simulink model "ARP_01_lib_TruthTables"  (R2014a)
settings: Solver=ode45  StartTime=0.0  StopTime=10.0  RelTol=1e-3
(part 2 of 2)

== stateflow chart ARP_01_lib_TruthTables/Chart ==
  note: num of bmlID=2
  note: num of bmlID=2
  note: num of bmlID=2
  note: num of sbmID=4
  note: num of bmlID=18
  note: num of bmlID=3
  note: num of bmlID=18
  note: num of bmlID=18
      | 17=neutralHead
      | 18=onceBlink
  note: num of bmlID=2
  note: num of bmlID=8
  note: num of bmlID=8
  data: bmlID function_input double; poseBML function_output double size=[256,1]; bmlID function_input double; poseBML function_output double size=[256,1]; bmlID function_input double; poseBML function_output double size=[256,1]; bmlID function_input double; poseBML function_output double size=[256,1]; bmlID function_input double; poseBML function_output double size=[256,1]; sbmID function_input double; poseSBM function_output double size=[256,1]; sbmID function_input double; poseSBM function_output double size=[256,1]; bmlID function_input double; poseBML function_output double size=[256,1]; bmlID function_input double; poseBML function_output double size=[256,1]; bmlID function_input double; poseBML function_output double size=[256,1]; bmlID function_input double; poseBML function_output double size=[256,1]; bmlID function_input double; gazeBML function_output double size=[256,1]; bmlID function_input double; gazeBML function_output double size=[256,1]; bmlID function_input double; poseBML function_output double size=[256,1]; bmlID function_input double; poseBML function_output double size=[256,1]; bmlID function_input double size=1; poseBML function_output double size=[256,1]; sbmID function_input double; poseSBM function_output double size=[256,1]; bmlID function_input double; poseBML function_output double size=[256,1]; bmlID function_input double; gazeBML function_output double size=[256,1]
  function poseBML = rockPoseTable(bmlID):
    | function poseBML = rockPoseTable(bmlID)
    | 
    | aVarTruthTableCondition_1 = false;
    | aVarTruthTableCondition_2 = false;
    | 
    | 
    | % rock
    | 
    | aVarTruthTableCondition_1 = logical(bmlID==1);
    | 
    | % rock
    | 
    | aVarTruthTableCondition_2 = logical(bmlID==2);
    | 
    | if (aVarTruthTableCondition_1)
    |     aFcnTruthTableAction_1();
    | elseif (aVarTruthTableCondition_2)
    |     aFcnTruthTableAction_2();
    | else % Default
    |     aFcnTruthTableAction_1();
    | end
    | 
    | function aFcnTruthTableAction_1()
    | 
    | % rock
    | 
    | poseBML=encStr2Arr('<?xml version="1.0" ?><act><bml><animation name="ChrBrad@Idle01_BeatFistMidLf02"/></bml></act>');
    | 
    | function aFcnTruthTableAction_2()
    | 
    | % rock2
    | 
    | poseBML=encStr2Arr('<?xml version="1.0" ?><act><bml><animation name="ChrBrad@Idle01_BeatFistMidLf01"/></bml></act>');
  function poseBML = paperPoseBradTable(bmlID):
    | function poseBML = paperPoseBradTable(bmlID)
    | 
    | aVarTruthTableCondition_1 = false;
    | aVarTruthTableCondition_2 = false;
    | 
    | 
    | % paper
    | 
    | aVarTruthTableCondition_1 = logical(bmlID==1);
    | 
    | % paper2
    | 
    | aVarTruthTableCondition_2 = logical(bmlID==2);
    | 
    | if (aVarTruthTableCondition_1)
    |     aFcnTruthTableAction_1();
    | elseif (aVarTruthTableCondition_2)
    |     aFcnTruthTableAction_2();
    | else % Default
    |     aFcnTruthTableAction_2();
    | end
    | 
    | function aFcnTruthTableAction_1()
    | 
    | % paper
    | 
    | poseBML=encStr2Arr('<?xml version="1.0" ?><act><bml><animation name="ChrBrad@Idle01_OfferLf01"/></bml></act>');
    | 
    | function aFcnTruthTableAction_2()
    | 
    | % paper2
    | 
    | poseBML=encStr2Arr('<?xml version="1.0" ?><act><bml><animation name="ChrBrad@Idle01_YouLf01"/></bml></act>');
  function poseBML = paperPoseRachelTable(bmlID):
    | function poseBML = paperPoseRachelTable(bmlID)
    | 
    | aVarTruthTableCondition_1 = false;
    | 
    | 
    | % paper
    | 
    | aVarTruthTableCondition_1 = logical(bmlID==1);
    | 
    | if (aVarTruthTableCondition_1)
    |     aFcnTruthTableAction_1();
    | else % Default
    |     aFcnTruthTableAction_1();
    | end
    | 
    | function aFcnTruthTableAction_1()
    | 
    | % paper
    | 
    | poseBML=encStr2Arr('<?xml version="1.0" ?><act><bml><animation name="ChrBrad@Idle01_YouLf01"/></bml></act>');
  function poseBML = scissorsPoseBradTable(bmlID):
    | function poseBML = scissorsPoseBradTable(bmlID)
    | 
    | aVarTruthTableCondition_1 = false;
    | aVarTruthTableCondition_2 = false;
    | 
    | 
    | % scissors
    | 
    | aVarTruthTableCondition_1 = logical(bmlID==1);
    | 
    | % scissors2
    | 
    | aVarTruthTableCondition_2 = logical(bmlID==2);
    | 
    | if (aVarTruthTableCondition_1)
    |     aFcnTruthTableAction_1();
    | elseif (aVarTruthTableCondition_2)
    |     aFcnTruthTableAction_2();
    | else % Default
    |     aFcnTruthTableAction_1();
    | end
    | 
    | function aFcnTruthTableAction_1()
    | 
    | % scissors
    | 
    | poseBML=encStr2Arr('<?xml version="1.0" ?><act><bml><animation name="ChrBrad@Idle01_YouLf01"/></bml></act>');
    | 
    | function aFcnTruthTableAction_2()
    | 
    | % scissors2
    | 
    | poseBML=encStr2Arr('<?xml version="1.0" ?><act><bml><animation name="ChrBrad@Idle01_OfferLf01"/></bml></act>');
  function poseBML = scissorsPoseRachelTable(bmlID):
    | function poseBML = scissorsPoseRachelTable(bmlID)
    | 
    | aVarTruthTableCondition_1 = false;
    | 
    | 
    | % scissors
    | 
    | aVarTruthTableCondition_1 = logical(bmlID==1);
    | 
    | if (aVarTruthTableCondition_1)
    |     aFcnTruthTableAction_1();
    | else % Default
    |     aFcnTruthTableAction_1();
    | end
    | 
    | function aFcnTruthTableAction_1()
    | 
    | % scissors
    | 
    | poseBML=encStr2Arr('<?xml version="1.0" ?><act><bml><animation name="ChrBrad@Idle01_YouLf01"/></bml></act>');
  function poseSBM = handPoseSBTable(sbmID):
    | function poseSBM = handPoseSBTable(sbmID)
    | 
    | aVarTruthTableCondition_1 = false;
    | aVarTruthTableCondition_2 = false;
    | aVarTruthTableCondition_3 = false;
    | aVarTruthTableCondition_4 = false;
    | 
    | 
    | % fingersClose
    | 
    | aVarTruthTableCondition_1 = logical(sbmID==1);
    | 
    | % fingersNeutral
    | 
    | aVarTruthTableCondition_2 = logical(sbmID==2);
    | 
    | % lshoulkderForward
    | 
    | aVarTruthTableCondition_3 = logical(sbmID==3);
    | 
    | % lshoulkderNeutral
    | 
    | aVarTruthTableCondition_4 = logical(sbmID==4);
    | 
    | if (aVarTruthTableCondition_1)
    |     aFcnTruthTableAction_1();
    | elseif (aVarTruthTableCondition_2)
    |     aFcnTruthTableAction_2();
    | elseif (aVarTruthTableCondition_3)
    |     aFcnTruthTableAction_3();
    | elseif (aVarTruthTableCondition_4)
    |     aFcnTruthTableAction_4();
    | else % Default
    |     aFcnTruthTableAction_1();
    | end
    | 
    | function aFcnTruthTableAction_1()
    | 
    | % fingersClose
    | 
    | poseSBM=encStr2Arr('brad.getSkeleton().getJointByName("l_pinky1").setPostrotation(SrQuat(1,0,0,0.5)); brad.getSkeleton().getJointByName("l_ring1").setPostrotation(SrQuat(1,0,0,0.5))');
    | 
    | function aFcnTruthTableAction_2()
    | 
    | % fingersNeutral
    | 
    | poseSBM=encStr2Arr('brad.getSkeleton().getJointByName("l_pinky1").setPostrotation(SrQuat(1,0,0,0)); brad.getSkeleton().getJointByName("l_ring1").setPostrotation(SrQuat(1,0,0,0))');
    | 
    | function aFcnTruthTableAction_3()
    | 
    | % lshoulkderForward
    | 
    | poseSBM=encStr2Arr('brad.getSkeleton().getJointByName("l_sternoclavicular").setPostrotation(SrQuat(1,0,0,0.05))');
    | 
    | function aFcnTruthTableAction_4()
    | 
    | % lshoulkderNeutral
    | 
    | poseSBM=encStr2Arr('brad.getSkeleton().getJointByName("l_sternoclavicular").setPostrotation(SrQuat(1,0,0,0))');
  function poseSBM = handPoseSBRachelTable(sbmID):
    | function poseSBM = handPoseSBRachelTable(sbmID)
    | 
    | aVarTruthTableCondition_1 = false;
    | aVarTruthTableCondition_2 = false;
    | aVarTruthTableCondition_3 = false;
    | aVarTruthTableCondition_4 = false;
    | 
    | 
    | % fingersClose
    | 
    | aVarTruthTableCondition_1 = logical(sbmID==1);
    | 
    | % fingersNeutral
    | 
    | aVarTruthTableCondition_2 = logical(sbmID==2);
    | 
    | % lshoulkderForward
    | 
    | aVarTruthTableCondition_3 = logical(sbmID==3);
    | 
    | % lshoulkderNeutral
    | 
    | aVarTruthTableCondition_4 = logical(sbmID==4);
    | 
    | if (aVarTruthTableCondition_1)
    |     aFcnTruthTableAction_1();
    | elseif (aVarTruthTableCondition_2)
    |     aFcnTruthTableAction_2();
    | elseif (aVarTruthTableCondition_3)
    |     aFcnTruthTableAction_3();
    | elseif (aVarTruthTableCondition_4)
    |     aFcnTruthTableAction_4();
    | else % Default
    |     aFcnTruthTableAction_1();
    | end
    | 
    | function aFcnTruthTableAction_1()
    | 
    | % fingersClose
    | 
    | poseSBM=encStr2Arr('Rachel.getSkeleton().getJointByName("l_pinky1").setPostrotation(SrQuat(1,0,0,0.5)); Rachel.getSkeleton().getJointByName("l_ring1").setPostrotation(SrQuat(1,0,0,0.5))');
    | 
    | function aFcnTruthTableAction_2()
    | 
    | % fingersNeutral
    | 
    | poseSBM=encStr2Arr('Rachel.getSkeleton().getJointByName("l_pinky1").setPostrotation(SrQuat(1,0,0,0)); Rachel.getSkeleton().getJointByName("l_ring1").setPostrotation(SrQuat(1,0,0,0))');
    | 
    | function aFcnTruthTableAction_3()
    | 
    | % lshoulkderForward
    | 
    | poseSBM=encStr2Arr('Rachel.getSkeleton().getJointByName("l_sternoclavicular").setPostrotation(SrQuat(1,0,0,0.05))');
    | 
    | function aFcnTruthTableAction_4()
    | 
    | % lshoulkderNeutral
    | 
    | poseSBM=encStr2Arr('Rachel.getSkeleton().getJointByName("l_sternoclavicular").setPostrotation(SrQuat(1,0,0,0))');
  function poseBML=idlePoseBradTable(bmlID):
    | function poseBML=idlePoseBradTable(bmlID)
    | 
    | aVarTruthTableCondition_1 = false;
    | aVarTruthTableCondition_2 = false;
    | aVarTruthTableCondition_3 = false;
    | aVarTruthTableCondition_4 = false;
    | aVarTruthTableCondition_5 = false;
    | aVarTruthTableCondition_6 = false;
    | aVarTruthTableCondition_7 = false;
    | aVarTruthTableCondition_8 = false;
    | aVarTruthTableCondition_9 = false;
    | aVarTruthTableCondition_10 = false;
    | aVarTruthTableCondition_11 = false;
    | aVarTruthTableCondition_12 = false;
    | aVarTruthTableCondition_13 = false;
    | aVarTruthTableCondition_14 = false;
    | aVarTruthTableCondition_15 = false;
    | aVarTruthTableCondition_16 = false;
    | aVarTruthTableCondition_17 = false;
    | aVarTruthTableCondition_18 = false;
    | 
    | 
    | 
    | aVarTruthTableCondition_1 = logical(bmlID==1);
    | 
    | 
    | aVarTruthTableCondition_2 = logical(bmlID==2);
    | 
    | 
    | aVarTruthTableCondition_3 = logical(bmlID==3);
    | 
    | 
    | aVarTruthTableCondition_4 = logical(bmlID==4);
    | 
    | 
    | aVarTruthTableCondition_5 = logical(bmlID==5);
    | 
    | 
    | aVarTruthTableCondition_6 = logical(bmlID==6);
    | 
    | 
    | aVarTruthTableCondition_7 = logical(bmlID==7);
    | 
    | 
    | aVarTruthTableCondition_8 = logical(bmlID==8);
    | 
    | 
    | aVarTruthTableCondition_9 = logical(bmlID==9);
    | 
    | 
    | aVarTruthTableCondition_10 = logical(bmlID==10);
    | 
    | 
    | aVarTruthTableCondition_11 = logical(bmlID==11);
    | 
    | 
    | aVarTruthTableCondition_12 = logical(bmlID==12);
    | 
    | 
    | aVarTruthTableCondition_13 = logical(bmlID==13);
    | 
    | 
    | aVarTruthTableCondition_14 = logical(bmlID==14);
    | 
    | 
    | aVarTruthTableCondition_15 = logical(bmlID==15);
    | 
    | 
    | aVarTruthTableCondition_16 = logical(bmlID==16);
    | 
    | 
    | aVarTruthTableCondition_17 = logical(bmlID==17);
    | 
    | 
    | aVarTruthTableCondition_18 = logical(bmlID==18);
    | 
    | if (aVarTruthTableCondition_1)
    |     aFcnTruthTableAction_1();
    | elseif (aVarTruthTableCondition_2)
    |     aFcnTruthTableAction_2();
    | elseif (aVarTruthTableCondition_3)
    |     aFcnTruthTableAction_3();
    | elseif (aVarTruthTableCondition_4)
    |     aFcnTruthTableAction_4();
    | elseif (aVarTruthTableCondition_5)
    |     aFcnTruthTableAction_5();
    | elseif (aVarTruthTableCondition_6)
    |     aFcnTruthTableAction_11();
    | elseif (aVarTruthTableCondition_7)
    |     aFcnTruthTableAction_3();
    | elseif (aVarTruthTableCondition_8)
    |     aFcnTruthTableAction_5();
    | elseif (aVarTruthTableCondition_9)
    |     aFcnTruthTableAction_3();
    | elseif (aVarTruthTableCondition_10)
    |     aFcnTruthTableAction_10();
    | elseif (aVarTruthTableCondition_11)
    |     aFcnTruthTableAction_11();
    | elseif (aVarTruthTableCondition_12)
    |     aFcnTruthTableAction_8();
    | elseif (aVarTruthTableCondition_13)
    |     aFcnTruthTableAction_8();
    | elseif (aVarTruthTableCondition_14)
    |     aFcnTruthTableAction_7();
    | elseif (aVarTruthTableCondition_15)
    |     aFcnTruthTableAction_6();
    | elseif (aVarTruthTableCondition_16)
    |     aFcnTruthTableAction_5();
    | elseif (aVarTruthTableCondition_17)
    |     aFcnTruthTableAction_8();
    | elseif (aVarTruthTableCondition_18)
    |     aFcnTruthTableAction_9();
    | else % Default
    |     aFcnTruthTableAction_3();
    | end
    | 
    | function aFcnTruthTableAction_1()
    | 
    | % ArmStretchHandsFW
    | 
    | poseBML=encStr2Arr('<?xml version="1.0" ?><act><bml><animation name="ChrBrad@Idle01_ArmStretch01"/></bml></act>');
    | 
    | function aFcnTruthTableAction_2()
    | 
    | % HandsOnWaist
    | 
    | poseBML=encStr2Arr('<?xml version="1.0" ?><act><bml><animation name="ChrBrad@Idle01_ToIdle03"/></bml></act>');
    | 
    | function aFcnTruthTableAction_3()
    | 
    | % WeightShift
    | 
    | poseBML=encStr2Arr('<?xml version="1.0" ?><act><bml><animation name="ChrBrad@Idle01_WeightShift01" /></bml></act>');
    | 
    | function aFcnTruthTableAction_4()
    | 
    | % ScratchChest
    | 
    | poseBML=encStr2Arr('<?xml version="1.0" ?><act><bml><animation name="ChrBrad@Idle01_ScratchChest01" /></bml></act>');
    | 
    | function aFcnTruthTableAction_5()
    | 
    | % ScratchHead
    | 
    | poseBML=encStr2Arr('<?xml version="1.0" ?><act><bml><animation name="ChrBrad@Idle01_ScratchHeadLf01" /></bml></act>');
    | 
    | function aFcnTruthTableAction_6()
    | 
    | % ShoulderStretchUpDown
    | 
    | poseBML=encStr2Arr('<?xml version="1.0" ?><act><bml><animation name="ChrBrad@Idle01_ShoulderStretch01" /></bml></act>');
    | 
    | function aFcnTruthTableAction_7()
    | 
    | % scratchtemple(head)
    | 
    | poseBML=encStr2Arr('<?xml version="1.0" ?><act><bml><animation name="ChrBrad@Idle01_ScratchTempleLf01" /></bml></act>');
    | 
    | function aFcnTruthTableAction_8()
    | 
    | % SqueezeHand01
    | 
    | poseBML=encStr2Arr('<?xml version="1.0" ?><act><bml><animation name="ChrBrad@Idle01_SqueezeHand01" /></bml></act>');
    | 
    | function aFcnTruthTableAction_9()
    | 
    | % TouchHands01
    | 
    | poseBML=encStr2Arr('<?xml version="1.0" ?><act><bml><animation name="ChrBrad@Idle01_TouchHands01" /></bml></act>');
    | 
    | function aFcnTruthTableAction_10()
    | 
    | % WeightShift2
    | 
    | poseBML=encStr2Arr('<?xml version="1.0" ?><act><bml><animation name="ChrBrad@Idle01_WeightShift02" /></bml></act>');
    | 
    | function aFcnTruthTableAction_11()
    | 
    | % Idle01_ToIdle02
    | 
    | poseBML=encStr2Arr('<?xml version="1.0" ?><act><bml><animation name="ChrBrad@Idle01_ToIdle02" /></bml></act>');
  function poseBML=initialPoseTable(bmlID):
    | function poseBML=initialPoseTable(bmlID)
    | 
    | aVarTruthTableCondition_1 = false;
    | aVarTruthTableCondition_2 = false;
    | aVarTruthTableCondition_3 = false;
    | 
    | 
    | 
    | aVarTruthTableCondition_1 = logical(bmlID==1);
    | 
    | 
    | aVarTruthTableCondition_2 = logical(bmlID==2);
    | 
    | 
    | aVarTruthTableCondition_3 = logical(bmlID==3);
    | 
    | if (aVarTruthTableCondition_1)
    |     aFcnTruthTableAction_1();
    | elseif (aVarTruthTableCondition_2)
    |     aFcnTruthTableAction_2();
    | elseif (aVarTruthTableCondition_3)
    |     aFcnTruthTableAction_3();
    | else % Default
    |     aFcnTruthTableAction_1();
    | end
    | 
    | function aFcnTruthTableAction_1()
    | 
    | % saccadeFinish
    | 
    | poseBML=encStr2Arr('<?xml version="1.0" ?><act><bml><saccade finish="true"/></bml></act>');
    | 
    | function aFcnTruthTableAction_2()
    | 
    | % neutralHeadGaze
    | 
    | poseBML=encStr2Arr('<?xml version="1.0" ?><act><bml><gaze target="camera" sbm:time-hint="0.2"/></bml></act>');
    | 
    | function aFcnTruthTableAction_3()
    | 
    | % blink
    | 
    | poseBML=encStr2Arr('<?xml version="1.0" ?><act><bml><face type="FACS" side="BOTH" au="45" amount="0.5" /></bml></act>');
  function poseBML=idlePoseRachelTable(bmlID):
    | function poseBML=idlePoseRachelTable(bmlID)
    | 
    | aVarTruthTableCondition_1 = false;
    | aVarTruthTableCondition_2 = false;
    | aVarTruthTableCondition_3 = false;
    | aVarTruthTableCondition_4 = false;
    | aVarTruthTableCondition_5 = false;
    | aVarTruthTableCondition_6 = false;
    | aVarTruthTableCondition_7 = false;
    | aVarTruthTableCondition_8 = false;
    | aVarTruthTableCondition_9 = false;
    | aVarTruthTableCondition_10 = false;
    | aVarTruthTableCondition_11 = false;
    | aVarTruthTableCondition_12 = false;
    | aVarTruthTableCondition_13 = false;
    | aVarTruthTableCondition_14 = false;
    | aVarTruthTableCondition_15 = false;
    | aVarTruthTableCondition_16 = false;
    | aVarTruthTableCondition_17 = false;
    | aVarTruthTableCondition_18 = false;
    | 
    | 
    | 
    | aVarTruthTableCondition_1 = logical(bmlID==1);
    | 
    | 
    | aVarTruthTableCondition_2 = logical(bmlID==2);
    | 
    | 
    | aVarTruthTableCondition_3 = logical(bmlID==3);
    | 
    | 
    | aVarTruthTableCondition_4 = logical(bmlID==4);
    | 
    | 
    | aVarTruthTableCondition_5 = logical(bmlID==5);
    | 
    | 
    | aVarTruthTableCondition_6 = logical(bmlID==6);
    | 
    | 
    | aVarTruthTableCondition_7 = logical(bmlID==7);
    | 
    | 
    | aVarTruthTableCondition_8 = logical(bmlID==8);
    | 
    | 
    | aVarTruthTableCondition_9 = logical(bmlID==9);
    | 
    | 
    | aVarTruthTableCondition_10 = logical(bmlID==10);
    | 
    | 
    | aVarTruthTableCondition_11 = logical(bmlID==11);
    | 
    | 
    | aVarTruthTableCondition_12 = logical(bmlID==12);
    | 
    | 
    | aVarTruthTableCondition_13 = logical(bmlID==13);
    | 
    | 
    | aVarTruthTableCondition_14 = logical(bmlID==14);
    | 
    | 
    | aVarTruthTableCondition_15 = logical(bmlID==15);
    | 
    | 
    | aVarTruthTableCondition_16 = logical(bmlID==16);
    | 
    | 
    | aVarTruthTableCondition_17 = logical(bmlID==17);
    | 
    | 
    | aVarTruthTableCondition_18 = logical(bmlID==18);
    | 
    | if (aVarTruthTableCondition_1)
    |     aFcnTruthTableAction_6();
    | elseif (aVarTruthTableCondition_2)
    |     aFcnTruthTableAction_2();
    | elseif (aVarTruthTableCondition_3)
    |     aFcnTruthTableAction_1();
    | elseif (aVarTruthTableCondition_4)
    |     aFcnTruthTableAction_2();
    | elseif (aVarTruthTableCondition_5)
    |     aFcnTruthTableAction_3();
    | elseif (aVarTruthTableCondition_6)
    |     aFcnTruthTableAction_7();
    | elseif (aVarTruthTableCondition_7)
    |     aFcnTruthTableAction_1();
    | elseif (aVarTruthTableCondition_8)
    |     aFcnTruthTableAction_3();
    | elseif (aVarTruthTableCondition_9)
    |     aFcnTruthTableAction_1();
    | elseif (aVarTruthTableCondition_10)
    |     aFcnTruthTableAction_6();
    | elseif (aVarTruthTableCondition_11)
    |     aFcnTruthTableAction_7();
    | elseif (aVarTruthTableCondition_12)
    |     aFcnTruthTableAction_5();
    | elseif (aVarTruthTableCondition_13)
    |     aFcnTruthTableAction_5();
    | elseif (aVarTruthTableCondition_14)
    |     aFcnTruthTableAction_3();
    | elseif (aVarTruthTableCondition_15)
    |     aFcnTruthTableAction_4();
    | elseif (aVarTruthTableCondition_16)
    |     aFcnTruthTableAction_3();
    | elseif (aVarTruthTableCondition_17)
    |     aFcnTruthTableAction_5();
    | elseif (aVarTruthTableCondition_18)
    |     aFcnTruthTableAction_3();
    | else % Default
    |     aFcnTruthTableAction_1();
    | end
    | 
    | function aFcnTruthTableAction_1()
    | 
    | % WeightShift
    | 
    | poseBML=encStr2Arr('<?xml version="1.0" ?><act><bml><animation name="ChrBrad@Idle01_WeightShift01" /></bml></act>');
    | 
    | function aFcnTruthTableAction_2()
    | 
    | % ScratchChest
    | 
    | poseBML=encStr2Arr('<?xml version="1.0" ?><act><bml><animation name="ChrRachel_ChrBrad@Idle01_ScratchChest01" /></bml></act>');
    | 
    | function aFcnTruthTableAction_3()
    | 
    | % ScratchHead
    | 
    | poseBML=encStr2Arr('<?xml version="1.0" ?><act><bml><animation name="ChrBrad@Idle01_ScratchHeadLf01" /></bml></act>');
    | 
    | function aFcnTruthTableAction_4()
    | 
    | % ShoulderStretchUpDown
    | 
    | poseBML=encStr2Arr('<?xml version="1.0" ?><act><bml><animation name="ChrBrad@Idle01_ShoulderStretch01" /></bml></act>');
    | 
    | function aFcnTruthTableAction_5()
    | 
    | % SqueezeHand01
    | 
    | poseBML=encStr2Arr('<?xml version="1.0" ?><act><bml><animation name="ChrBrad@Idle01_SqueezeHand01" /></bml></act>');
    | 
    | function aFcnTruthTableAction_6()
    | 
    | % WeightShift2
    | 
    | poseBML=encStr2Arr('<?xml version="1.0" ?><act><bml><animation name="ChrBrad@Idle01_WeightShift02" /></bml></act>');
    | 
    | function aFcnTruthTableAction_7()
    | 
    | % Idle01_ToIdle02
    | 
    | poseBML=encStr2Arr('<?xml version="1.0" ?><act><bml><animation name="ChrBrad@Idle01_ToIdle02" /></bml></act>');
  function poseBML = successTable(bmlID):
    | function poseBML = successTable(bmlID)
    | 
    | aVarTruthTableCondition_1 = false;
    | aVarTruthTableCondition_2 = false;
    | aVarTruthTableCondition_3 = false;
    | 
    | 
    | % smile
    | 
    | aVarTruthTableCondition_1 = logical(bmlID==1);
    | 
    | % HeadChestUp
    | 
    | aVarTruthTableCondition_2 = logical(bmlID==2);
    | 
    | % browUp
    | 
    | aVarTruthTableCondition_3 = logical(bmlID==3);
    | 
    | if (aVarTruthTableCondition_1)
    |     aFcnTruthTableAction_1();
    | elseif (aVarTruthTableCondition_2)
    |     aFcnTruthTableAction_2();
    | elseif (aVarTruthTableCondition_3)
    |     aFcnTruthTableAction_3();
    | else % Default
    |     aFcnTruthTableAction_1();
    | end
    | 
    | function aFcnTruthTableAction_1()
    | 
    | % smile
    | 
    | poseBML=encStr2Arr('<?xml version="1.0" ?><act><bml><face amount="1" au="12" end="8" relax="6" side="BOTH" start="0" stroke="3" type="facs"/><face amount="0.5" au="6" end="8" relax="6" side="BOTH" start="0" stroke="3" type="facs"/></bml></act>');
    | 
    | function aFcnTruthTableAction_2()
    | 
    | % HeadChestUp
    | 
    | poseBML=encStr2Arr('<?xml version="1.0" ?><act><bml><gaze angle="12" direction="UP" sbm:joint-range="HEAD CHEST" sbm:time-hint="0.3" target="camera"/></bml></act>');
    | 
    | function aFcnTruthTableAction_3()
    | 
    | % browUp
    | 
    | poseBML=encStr2Arr('<?xml version="1.0" ?><act><bml><face amount="0.3" au="1" end="6" side="BOTH" start="0" type="facs"/><face amount="0.8"  au="2" end="6" side="BOTH" start="0" type="facs"/></bml></act>');
  function gazeBML=idleGazeNotInterestedTable(bmlID):
    | function gazeBML=idleGazeNotInterestedTable(bmlID)
    | 
    | aVarTruthTableCondition_1 = false;
    | aVarTruthTableCondition_2 = false;
    | aVarTruthTableCondition_3 = false;
    | aVarTruthTableCondition_4 = false;
    | aVarTruthTableCondition_5 = false;
    | aVarTruthTableCondition_6 = false;
    | aVarTruthTableCondition_7 = false;
    | aVarTruthTableCondition_8 = false;
    | aVarTruthTableCondition_9 = false;
    | aVarTruthTableCondition_10 = false;
    | aVarTruthTableCondition_11 = false;
    | aVarTruthTableCondition_12 = false;
    | aVarTruthTableCondition_13 = false;
    | aVarTruthTableCondition_14 = false;
    | aVarTruthTableCondition_15 = false;
    | aVarTruthTableCondition_16 = false;
    | aVarTruthTableCondition_17 = false;
    | aVarTruthTableCondition_18 = false;
    | 
    | 
    | 
    | aVarTruthTableCondition_1 = logical(bmlID==1);
    | 
    | 
    | aVarTruthTableCondition_2 = logical(bmlID==2);
    | 
    | 
    | aVarTruthTableCondition_3 = logical(bmlID==3);
    | 
    | 
    | aVarTruthTableCondition_4 = logical(bmlID==4);
    | 
    | 
    | aVarTruthTableCondition_5 = logical(bmlID==5);
    | 
    | 
    | aVarTruthTableCondition_6 = logical(bmlID==6);
    | 
    | 
    | aVarTruthTableCondition_7 = logical(bmlID==7);
    | 
    | 
    | aVarTruthTableCondition_8 = logical(bmlID==8);
    | 
    | 
    | aVarTruthTableCondition_9 = logical(bmlID==9);
    | 
    | 
    | aVarTruthTableCondition_10 = logical(bmlID==10);
    | 
    | 
    | aVarTruthTableCondition_11 = logical(bmlID==11);
    | 
    | 
    | aVarTruthTableCondition_12 = logical(bmlID==12);
    | 
    | 
    | aVarTruthTableCondition_13 = logical(bmlID==13);
    | 
    | 
    | aVarTruthTableCondition_14 = logical(bmlID==14);
    | 
    | 
    | aVarTruthTableCondition_15 = logical(bmlID==15);
    | 
    | 
    | aVarTruthTableCondition_16 = logical(bmlID==16);
    | 
    | 
    | aVarTruthTableCondition_17 = logical(bmlID==17);
    | 
    | 
    | aVarTruthTableCondition_18 = logical(bmlID==18);
    | 
    | if (aVarTruthTableCondition_1)
    |     aFcnTruthTableAction_1();
    | elseif (aVarTruthTableCondition_2)
    |     aFcnTruthTableAction_2();
    | elseif (aVarTruthTableCondition_3)
    |     aFcnTruthTableAction_3();
    | elseif (aVarTruthTableCondition_4)
    |     aFcnTruthTableAction_4();
    | elseif (aVarTruthTableCondition_5)
    |     aFcnTruthTableAction_5();
    | elseif (aVarTruthTableCondition_6)
    |     aFcnTruthTableAction_6();
    | elseif (aVarTruthTableCondition_7)
    |     aFcnTruthTableAction_7();
    | elseif (aVarTruthTableCondition_8)
    |     aFcnTruthTableAction_8();
    | elseif (aVarTruthTableCondition_9)
    |     aFcnTruthTableAction_9();
    | elseif (aVarTruthTableCondition_10)
    |     aFcnTruthTableAction_10();
    | elseif (aVarTruthTableCondition_11)
    |     aFcnTruthTableAction_11();
    | elseif (aVarTruthTableCondition_12)
    |     aFcnTruthTableAction_12();
    | elseif (aVarTruthTableCondition_13)
    |     aFcnTruthTableAction_13();
    | elseif (aVarTruthTableCondition_14)
    |     aFcnTruthTableAction_14();
    | elseif (aVarTruthTableCondition_15)
    |     aFcnTruthTableAction_15();
    | elseif (aVarTruthTableCondition_16)
    |     aFcnTruthTableAction_16();
    | elseif (aVarTruthTableCondition_17)
    |     aFcnTruthTableAction_17();
    | elseif (aVarTruthTableCondition_18)
    |     aFcnTruthTableAction_18();
    | else % Default
    |     aFcnTruthTableAction_1();
    | end
    | 
    | function aFcnTruthTableAction_1()
    | 
    | % LeftS
    | 
    | gazeBML=encStr2Arr('<?xml version="1.0" ?><act><bml><gaze angle="12" direction="LEFT" sbm:joint-range="EYES" target="camera"/></bml></act>');
    | 
    | function aFcnTruthTableAction_2()
    | 
    | % RightS
    | 
    | gazeBML=encStr2Arr('<?xml version="1.0" ?><act><bml><gaze angle="12" direction="RIGHT" sbm:joint-range="EYES" target="camera"/></bml></act>');
    | 
    | function aFcnTruthTableAction_3()
    | 
    | % UpS
    | 
    | gazeBML=encStr2Arr('<?xml version="1.0" ?><act><bml><gaze angle="12" direction="UP" sbm:joint-range="EYES" target="camera"/></bml></act>');
    | 
    | function aFcnTruthTableAction_4()
    | 
    | % DownS
    | 
    | gazeBML=encStr2Arr('<?xml version="1.0" ?><act><bml><gaze angle="12" direction="DOWN" sbm:joint-range="EYES" target="camera"/></bml></act>');
    | 
    | function aFcnTruthTableAction_5()
    | 
    | % UpLeftS
    | 
    | gazeBML=encStr2Arr('<?xml version="1.0" ?><act><bml><gaze angle="12" direction="UPLEFT" sbm:joint-range="EYES" target="camera"/></bml></act>');
    | 
    | function aFcnTruthTableAction_6()
    | 
    | % UpRightS
    | 
    | gazeBML=encStr2Arr('<?xml version="1.0" ?><act><bml><gaze angle="12" direction="UPRIGHT" sbm:joint-range="EYES" target="camera"/></bml></act>');
    | 
    | function aFcnTruthTableAction_7()
    | 
    | % DownLeftS
    | 
    | gazeBML=encStr2Arr('<?xml version="1.0" ?><act><bml><gaze angle="12" direction="DOWNLEFT" sbm:joint-range="EYES" target="camera"/></bml></act>');
    | 
    | function aFcnTruthTableAction_8()
    | 
    | % DownRightS
    | 
    | gazeBML=encStr2Arr('<?xml version="1.0" ?><act><bml><gaze angle="12" direction="DOWNRIGHT" sbm:joint-range="EYES" target="camera"/></bml></act>');
    | 
    | function aFcnTruthTableAction_9()
    | 
    | % Down
    | 
    | gazeBML=encStr2Arr('<?xml version="1.0" ?><act><bml><gaze direction="DOWN" sbm:joint-range="EYES NECK" sbm:time-hint="0.15" target="camera"/></bml></act>');
    | 
    | function aFcnTruthTableAction_10()
    | 
    | % Downleft
    | 
    | gazeBML=encStr2Arr('<?xml version="1.0" ?><act><bml><gaze direction="DOWNLEFT" sbm:joint-range="EYES NECK" sbm:time-hint="0.15" target="camera"/></bml></act>');
    | 
    | function aFcnTruthTableAction_11()
    | 
    | % Downright
    | 
    | gazeBML=encStr2Arr('<?xml version="1.0" ?><act><bml><gaze direction="DOWNRIGHT" sbm:joint-range="EYES NECK" sbm:time-hint="0.15" target="camera"/></bml></act>');
    | 
    | function aFcnTruthTableAction_12()
    | 
    | % Upright
    | 
    | gazeBML=encStr2Arr('<?xml version="1.0" ?><act><bml><gaze direction="UPRIGHT" sbm:joint-range="EYES NECK" sbm:time-hint="0.15" target="camera"/></bml></act>');
    | 
    | function aFcnTruthTableAction_13()
    | 
    | % Upleft
    | 
    | gazeBML=encStr2Arr('<?xml version="1.0" ?><act><bml><gaze direction="UPLEFT" sbm:joint-range="EYES NECK" sbm:time-hint="0.15" target="camera"/></bml></act>');
    | 
    | function aFcnTruthTableAction_14()
    | 
    | % Up
    | 
    | gazeBML=encStr2Arr('<?xml version="1.0" ?><act><bml><gaze direction="UP" sbm:joint-range="EYES NECK" sbm:time-hint="0.15" target="camera"/></bml></act>');
    | 
    | function aFcnTruthTableAction_15()
    | 
    | % Right
    | 
    | gazeBML=encStr2Arr('<?xml version="1.0" ?><act><bml><gaze direction="RIGHT" sbm:joint-range="EYES NECK" sbm:time-hint="0.15" target="camera"/></bml></act>');
    | 
    | function aFcnTruthTableAction_16()
    | 
    | % LEFT
    | 
    | gazeBML=encStr2Arr('<?xml version="1.0" ?><act><bml><gaze direction="LEFT" sbm:joint-range="EYES NECK" sbm:time-hint="0.15" target="camera"/></bml></act>');
    | 
    | function aFcnTruthTableAction_17()
    | 
    | % neutralHeadGaze
    | 
    | gazeBML=encStr2Arr('<?xml version="1.0" ?><act><bml><gaze target="camera" sbm:time-hint="0.2"/></bml></act>');
    | 
    | function aFcnTruthTableAction_18()
    | 
    | % blinkOnce
    | 
    | poseBML=encStr2Arr('<?xml version="1.0" ?><act><bml><face type="FACS" side="BOTH" au="45" start="0" end="0.1" amount="1" /></bml></act>');
  function gazeBML=idleGazeInterestedTable(bmlID):
    | function gazeBML=idleGazeInterestedTable(bmlID)
    | 
    | aVarTruthTableCondition_1 = false;
    | aVarTruthTableCondition_2 = false;
    | aVarTruthTableCondition_3 = false;
    | aVarTruthTableCondition_4 = false;
    | aVarTruthTableCondition_5 = false;
    | aVarTruthTableCondition_6 = false;
    | aVarTruthTableCondition_7 = false;
    | 
    | 
    | 
    | aVarTruthTableCondition_1 = logical(bmlID==1);
    | 
    | 
    | aVarTruthTableCondition_2 = logical(bmlID==2);
    | 
    | 
    | aVarTruthTableCondition_3 = logical(bmlID==3);
    | 
    | 
    | aVarTruthTableCondition_4 = logical(bmlID==4);
    | 
    | 
    | aVarTruthTableCondition_5 = logical(bmlID==5);
    | 
    | 
    | aVarTruthTableCondition_6 = logical(bmlID==6);
    | 
    | 
    | aVarTruthTableCondition_7 = logical(bmlID==7);
    | 
    | if (aVarTruthTableCondition_1)
    |     aFcnTruthTableAction_1();
    | elseif (aVarTruthTableCondition_2)
    |     aFcnTruthTableAction_2();
    | elseif (aVarTruthTableCondition_3)
    |     aFcnTruthTableAction_3();
    | elseif (aVarTruthTableCondition_4)
    |     aFcnTruthTableAction_4();
    | elseif (aVarTruthTableCondition_5)
    |     aFcnTruthTableAction_5();
    | elseif (aVarTruthTableCondition_6)
    |     aFcnTruthTableAction_6();
    | elseif (aVarTruthTableCondition_7)
    |     aFcnTruthTableAction_7();
    | else % Default
    |     aFcnTruthTableAction_1();
    | end
    | 
    | function aFcnTruthTableAction_1()
    | 
    | % UpS
    | 
    | gazeBML=encStr2Arr('<?xml version="1.0" ?><act><bml><gaze angle="5" direction="UP" sbm:joint-range="EYES" target="camera"/></bml></act>');
    | 
    | function aFcnTruthTableAction_2()
    | 
    | % DownS
    | 
    | gazeBML=encStr2Arr('<?xml version="1.0" ?><act><bml><gaze angle="5" direction="DOWN" sbm:joint-range="EYES" target="camera"/></bml></act>');
    | 
    | function aFcnTruthTableAction_3()
    | 
    | % DownS
    | 
    | gazeBML=encStr2Arr('<?xml version="1.0" ?><act><bml><gaze angle="10" direction="DOWN" sbm:joint-range="EYES" target="camera"/></bml></act>');
    | 
    | function aFcnTruthTableAction_4()
    | 
    | % UpLeftS
    | 
    | gazeBML=encStr2Arr('<?xml version="1.0" ?><act><bml><gaze angle="3" direction="UPLEFT" sbm:joint-range="EYES" target="camera"/></bml></act>');
    | 
    | function aFcnTruthTableAction_5()
    | 
    | % UpRightS
    | 
    | gazeBML=encStr2Arr('<?xml version="1.0" ?><act><bml><gaze angle="3" direction="UPRIGHT" sbm:joint-range="EYES" target="camera"/></bml></act>');
    | 
    | function aFcnTruthTableAction_6()
    | 
    | % DownLeftS
    | 
    | gazeBML=encStr2Arr('<?xml version="1.0" ?><act><bml><gaze angle="3" direction="DOWNLEFT" sbm:joint-range="EYES" target="camera"/></bml></act>');
    | 
    | function aFcnTruthTableAction_7()
    | 
    | % DownRightS
    | 
    | gazeBML=encStr2Arr('<?xml version="1.0" ?><act><bml><gaze angle="3" direction="DOWNRIGHT" sbm:joint-range="EYES" target="camera"/></bml></act>');
  function poseBML = smileTable(bmlID):
    | function poseBML = smileTable(bmlID)
    | 
    | aVarTruthTableCondition_1 = false;
    | aVarTruthTableCondition_2 = false;
    | 
    | 
    | % smile
    | 
    | aVarTruthTableCondition_1 = logical(bmlID==2);
    | 
    | % neutralHeadGaze
    | 
    | aVarTruthTableCondition_2 = logical(bmlID==3);
    | 
    | if (aVarTruthTableCondition_1)
    |     aFcnTruthTableAction_1();
    | elseif (aVarTruthTableCondition_2)
    |     aFcnTruthTableAction_2();
    | else % Default
    |     aFcnTruthTableAction_1();
    | end
    | 
    | function aFcnTruthTableAction_1()
    | 
    | % smile
    | 
    | poseBML=encStr2Arr('<?xml version="1.0" ?><act><bml><face amount="1" au="12" end="8" relax="6" side="BOTH" start="0" stroke="3" type="facs"/><face amount="0.5" au="6" end="8" relax="6" side="BOTH" start="0" stroke="3" type="facs"/></bml></act>');
    | 
    | function aFcnTruthTableAction_2()
    | 
    | % neutralHeadGaze
    | 
    | poseBML=encStr2Arr('<?xml version="1.0" ?><act><bml><gaze target="camera" sbm:time-hint="0.2"/></bml></act>');
  function poseBML=idlePoseBradSTable(bmlID):
    | function poseBML=idlePoseBradSTable(bmlID)
    | 
    | aVarTruthTableCondition_1 = false;
    | aVarTruthTableCondition_2 = false;
    | aVarTruthTableCondition_3 = false;
    | aVarTruthTableCondition_4 = false;
    | aVarTruthTableCondition_5 = false;
    | aVarTruthTableCondition_6 = false;
    | aVarTruthTableCondition_7 = false;
    | aVarTruthTableCondition_8 = false;
    | 
    | 
    | 
    | aVarTruthTableCondition_1 = logical(bmlID==1);
    | 
    | 
    | aVarTruthTableCondition_2 = logical(bmlID==2);
    | 
    | 
    | aVarTruthTableCondition_3 = logical(bmlID==3);
    | 
    | 
    | aVarTruthTableCondition_4 = logical(bmlID==4);
    | 
    | 
    | aVarTruthTableCondition_5 = logical(bmlID==5);
    | 
    | 
    | aVarTruthTableCondition_6 = logical(bmlID==6);
    | 
    | 
    | aVarTruthTableCondition_7 = logical(bmlID==7);
    | 
    | 
    | aVarTruthTableCondition_8 = logical(bmlID==8);
    | 
    | if (aVarTruthTableCondition_1)
    |     aFcnTruthTableAction_1();
    | elseif (aVarTruthTableCondition_2)
    |     aFcnTruthTableAction_2();
    | elseif (aVarTruthTableCondition_3)
    |     aFcnTruthTableAction_3();
    | elseif (aVarTruthTableCondition_4)
    |     aFcnTruthTableAction_4();
    | elseif (aVarTruthTableCondition_5)
    |     aFcnTruthTableAction_5();
    | elseif (aVarTruthTableCondition_6)
    |     aFcnTruthTableAction_6();
    | elseif (aVarTruthTableCondition_7)
    |     aFcnTruthTableAction_3();
    | elseif (aVarTruthTableCondition_8)
    |     aFcnTruthTableAction_5();
    | else % Default
    |     aFcnTruthTableAction_3();
    | end
    | 
    | function aFcnTruthTableAction_1()
    | 
    | % ArmStretch
    | 
    | poseBML=encStr2Arr('<?xml version="1.0" ?><act><bml><animation name="ChrBrad@Idle01_ArmStretch01" start="0" end="1"/></bml></act>')
    | 
    | function aFcnTruthTableAction_2()
    | 
    | % Idle01_ToIdle03
    | 
    | poseBML=encStr2Arr('<?xml version="1.0" ?><act><bml><animation name="ChrBrad@Idle01_ToIdle03" start="0" end="1"/></bml></act>')
    | 
    | function aFcnTruthTableAction_3()
    | 
    | % WeightShift
    | 
    | poseBML=encStr2Arr('<?xml version="1.0" ?><act><bml><animation name="ChrBrad@Idle01_WeightShift01" start="0" end="2"/></bml></act>')
    | 
    | function aFcnTruthTableAction_4()
    | 
    | % ScratchChest
    | 
    | poseBML=encStr2Arr('<?xml version="1.0" ?><act><bml><animation name="ChrBrad@Idle01_ScratchChest01" start="0" end="1"/></bml></act>')
    | 
    | function aFcnTruthTableAction_5()
    | 
    | % ScratchHead
    | 
    | poseBML=encStr2Arr('<?xml version="1.0" ?><act><bml><animation name="ChrBrad@Idle01_ScratchHeadLf01" start="0" end="1"/></bml></act>')
    | 
    | function aFcnTruthTableAction_6()
    | 
    | % ShoulderStretch
    | 
    | poseBML=encStr2Arr('<?xml version="1.0" ?><act><bml><animation name="ChrBrad@Idle01_ShoulderStretch01" start="0" end="1"/></bml></act>')
  function poseBML=idlePoseRachelSTable(bmlID):
    | function poseBML=idlePoseRachelSTable(bmlID)
    | 
    | aVarTruthTableCondition_1 = false;
    | aVarTruthTableCondition_2 = false;
    | aVarTruthTableCondition_3 = false;
    | aVarTruthTableCondition_4 = false;
    | aVarTruthTableCondition_5 = false;
    | aVarTruthTableCondition_6 = false;
    | aVarTruthTableCondition_7 = false;
    | aVarTruthTableCondition_8 = false;
    | 
    | 
    | 
    | aVarTruthTableCondition_1 = logical(bmlID==1);
    | 
    | 
    | aVarTruthTableCondition_2 = logical(bmlID==2);
    | 
    | 
    | aVarTruthTableCondition_3 = logical(bmlID==3);
    | 
    | 
    | aVarTruthTableCondition_4 = logical(bmlID==4);
    | 
    | 
    | aVarTruthTableCondition_5 = logical(bmlID==5);
    | 
    | 
    | aVarTruthTableCondition_6 = logical(bmlID==6);
    | 
    | 
    | aVarTruthTableCondition_7 = logical(bmlID==7);
    | 
    | 
    | aVarTruthTableCondition_8 = logical(bmlID==8);
    | 
    | if (aVarTruthTableCondition_1)
    |     aFcnTruthTableAction_1();
    | elseif (aVarTruthTableCondition_2)
    |     aFcnTruthTableAction_2();
    | elseif (aVarTruthTableCondition_3)
    |     aFcnTruthTableAction_3();
    | elseif (aVarTruthTableCondition_4)
    |     aFcnTruthTableAction_4();
    | elseif (aVarTruthTableCondition_5)
    |     aFcnTruthTableAction_5();
    | elseif (aVarTruthTableCondition_6)
    |     aFcnTruthTableAction_6();
    | elseif (aVarTruthTableCondition_7)
    |     aFcnTruthTableAction_3();
    | elseif (aVarTruthTableCondition_8)
    |     aFcnTruthTableAction_5();
    | else % Default
    |     aFcnTruthTableAction_3();
    | end
    | 
    | function aFcnTruthTableAction_1()
    | 
    | % ArmStretch
    | 
    | poseBML=encStr2Arr('<?xml version="1.0" ?><act><bml><animation name="ChrRachel_ChrBrad@Idle01_ArmStretch01" start="0" end="1"/></bml></act>')
    | 
    | function aFcnTruthTableAction_2()
    | 
    | % Idle01_ToIdle03
    | 
    | poseBML=encStr2Arr('<?xml version="1.0" ?><act><bml><animation name="ChrRachel_ChrBrad@Idle01_ToIdle03" start="0" end="1"/></bml></act>')
    | 
    | function aFcnTruthTableAction_3()
    | 
    | % WeightShift
    | 
    | poseBML=encStr2Arr('<?xml version="1.0" ?><act><bml><animation name="ChrRachel_ChrBrad@Idle01_WeightShift01" start="0" end="2"/></bml></act>')
    | 
    | function aFcnTruthTableAction_4()
    | 
    | % ScratchChest
    | 
    | poseBML=encStr2Arr('<?xml version="1.0" ?><act><bml><animation name="ChrRachel_ChrBrad@Idle01_ScratchChest01" start="0" end="1"/></bml></act>')
    | 
    | function aFcnTruthTableAction_5()
    | 
    | % ScratchHead
    | 
    | poseBML=encStr2Arr('<?xml version="1.0" ?><act><bml><animation name="ChrRachel_ChrBrad@Idle01_ScratchHeadLf01" start="0" end="1"/></bml></act>')
    | 
    | function aFcnTruthTableAction_6()
    | 
    | % ShoulderStretch
    | 
    | poseBML=encStr2Arr('<?xml version="1.0" ?><act><bml><animation name="ChrRachel_ChrBrad@Idle01_ShoulderStretch01" start="0" end="1"/></bml></act>')
  function poseSBM = handPoseSBCompleteTable(sbmID):
    | function poseSBM = handPoseSBCompleteTable(sbmID)
    | 
    | aVarTruthTableCondition_1 = false;
    | aVarTruthTableCondition_2 = false;
    | aVarTruthTableCondition_3 = false;
    | aVarTruthTableCondition_4 = false;
    | aVarTruthTableCondition_5 = false;
    | aVarTruthTableCondition_6 = false;
    | 
    | 
    | % fingersClose
    | 
    | aVarTruthTableCondition_1 = logical(sbmID==1);
    | 
    | % fingersNeutral
    | 
    | aVarTruthTableCondition_2 = logical(sbmID==2);
    | 
    | % lshoulkderForward
    | 
    | aVarTruthTableCondition_3 = logical(sbmID==3);
    | 
    | % lshoulkderNeutral
    | 
    | aVarTruthTableCondition_4 = logical(sbmID==4);
    | 
    | % lwristRotate
    | 
    | aVarTruthTableCondition_5 = logical(sbmID==5);
    | 
    | % lwristNeutral
    | 
    | aVarTruthTableCondition_6 = logical(sbmID==6);
    | 
    | if (aVarTruthTableCondition_1)
    |     aFcnTruthTableAction_1();
    | elseif (aVarTruthTableCondition_2)
    |     aFcnTruthTableAction_2();
    | elseif (aVarTruthTableCondition_3)
    |     aFcnTruthTableAction_3();
    | elseif (aVarTruthTableCondition_4)
    |     aFcnTruthTableAction_4();
    | elseif (aVarTruthTableCondition_5)
    |     aFcnTruthTableAction_5();
    | elseif (aVarTruthTableCondition_6)
    |     aFcnTruthTableAction_6();
    | else % Default
    |     aFcnTruthTableAction_6();
    | end
    | 
    | function aFcnTruthTableAction_1()
    | 
    | % fingersClose
    | 
    | poseSBM=encStr2Arr('brad.getSkeleton().getJointByName("l_pinky1").setPostrotation(SrQuat(1,0,0,0.5)); brad.getSkeleton().getJointByName("l_ring1").setPostrotation(SrQuat(1,0,0,0.5))')
    | 
    | function aFcnTruthTableAction_2()
    | 
    | % fingersNeutral
    | 
    | poseSBM=encStr2Arr('brad.getSkeleton().getJointByName("l_pinky1").setPostrotation(SrQuat(1,0,0,0)); brad.getSkeleton().getJointByName("l_ring1").setPostrotation(SrQuat(1,0,0,0))')
    | 
    | function aFcnTruthTableAction_3()
    | 
    | % lshoulkderForward
    | 
    | poseSBM=encStr2Arr('brad.getSkeleton().getJointByName("l_sternoclavicular").setPostrotation(SrQuat(1,0,0,0.05));')
    | 
    | function aFcnTruthTableAction_4()
    | 
    | % lshoulkderNeutral
    | 
    | poseSBM=encStr2Arr('brad.getSkeleton().getJointByName("l_sternoclavicular").setPostrotation(SrQuat(1,0,0,0));')
    | 
    | function aFcnTruthTableAction_5()
    | 
    | % lwristRotate
    | 
    | poseSBM=encStr2Arr('brad.getSkeleton().getJointByName("l_wrist").setPostrotation(SrQuat(-1,0.1,0,0));')
    | 
    | function aFcnTruthTableAction_6()
    | 
    | % lwristNeutral
    | 
    | poseSBM=encStr2Arr('brad.getSkeleton().getJointByName("l_wrist").setPostrotation(SrQuat(1,0,0,0));')
  function poseBML = idlePoseCompleteTable(bmlID):
    | function poseBML = idlePoseCompleteTable(bmlID)
    | 
    | aVarTruthTableCondition_1 = false;
    | aVarTruthTableCondition_2 = false;
    | aVarTruthTableCondition_3 = false;
    | aVarTruthTableCondition_4 = false;
    | aVarTruthTableCondition_5 = false;
    | aVarTruthTableCondition_6 = false;
    | aVarTruthTableCondition_7 = false;
    | aVarTruthTableCondition_8 = false;
    | 
    | 
    | % nolean
    | 
    | aVarTruthTableCondition_1 = logical(bmlID==1);
    | 
    | % lean
    | 
    | aVarTruthTableCondition_2 = logical(bmlID==2);
    | 
    | % gaze
    | 
    | aVarTruthTableCondition_3 = logical(bmlID==3);
    | 
    | % smile
    | 
    | aVarTruthTableCondition_4 = logical(bmlID==4);
    | 
    | % smile5
    | 
    | aVarTruthTableCondition_5 = logical(bmlID==5);
    | 
    | % smile7
    | 
    | aVarTruthTableCondition_6 = logical(bmlID==6);
    | 
    | % smile10
    | 
    | aVarTruthTableCondition_7 = logical(bmlID==7);
    | 
    | % neutralHeadGaze
    | 
    | aVarTruthTableCondition_8 = logical(bmlID==8);
    | 
    | if (aVarTruthTableCondition_1)
    |     aFcnTruthTableAction_1();
    | elseif (aVarTruthTableCondition_2)
    |     aFcnTruthTableAction_2();
    | elseif (aVarTruthTableCondition_3)
    |     aFcnTruthTableAction_3();
    | elseif (aVarTruthTableCondition_4)
    |     aFcnTruthTableAction_4();
    | elseif (aVarTruthTableCondition_5)
    |     aFcnTruthTableAction_5();
    | elseif (aVarTruthTableCondition_6)
    |     aFcnTruthTableAction_6();
    | elseif (aVarTruthTableCondition_7)
    |     aFcnTruthTableAction_7();
    | elseif (aVarTruthTableCondition_8)
    |     aFcnTruthTableAction_8();
    | else % Default
    |     aFcnTruthTableAction_8();
    | end
    | 
    | function aFcnTruthTableAction_1()
    | 
    | % nolean
    | 
    | poseBML=encStr2Arr('<?xml version="1.0" ?><act><bml><gaze sbm:joint-range="EYES BACK" target="camera"/><gaze sbm:joint-range="CHEST BACK" target="camera"/></bml></act>')
    | 
    | function aFcnTruthTableAction_2()
    | 
    | % lean
    | 
    | poseBML=encStr2Arr('<?xml version="1.0" ?><act><bml><gaze sbm:joint-range="EYES BACK" target="camera"/><gaze direction="DOWN" sbm:joint-range="CHEST BACK" target="camera"/></bml></act>')
    | 
    | function aFcnTruthTableAction_3()
    | 
    | % gaze
    | 
    | poseBML=encStr2Arr('<?xml version="1.0" ?><act><bml><saccade finish="true"/></bml></act>')
    | 
    | function aFcnTruthTableAction_4()
    | 
    | % smile
    | 
    | poseBML=encStr2Arr('<?xml version="1.0" ?><act><bml><face amount="1" au="12" end="8" relax="6" side="BOTH" start="0" stroke="3" type="facs"/><face amount="0.5" au="6" end="8" relax="6" side="BOTH" start="0" stroke="3" type="facs"/></bml></act>')
    | 
    | function aFcnTruthTableAction_5()
    | 
    | % smile5
    | 
    | poseBML=encStr2Arr('<?xml version="1.0" ?><act><bml><face amount="1" au="12" end="9" relax="7" side="BOTH" start="0" stroke="3" type="facs"/><face amount="0.5" au="6" end="9" relax="7" side="BOTH" start="0" stroke="3" type="facs"/></bml></act>')
    | 
    | function aFcnTruthTableAction_6()
    | 
    | % smile7
    | 
    | poseBML=encStr2Arr('<?xml version="1.0" ?><act><bml><face amount="1" au="12" end="10" relax="8" side="BOTH" start="0" stroke="3" type="facs"/><face amount="0.5" au="6" end="10" relax="8" side="BOTH" start="0" stroke="3" type="facs"/></bml></act>')
    | 
    | function aFcnTruthTableAction_7()
    | 
    | % smile10
    | 
    | poseBML=encStr2Arr('<?xml version="1.0" ?><act><bml><face amount="1" au="12" end="11" relax="9" side="BOTH" start="0" stroke="3" type="facs"/><face amount="0.5" au="6" end="11" relax="9" side="BOTH" start="0" stroke="3" type="facs"/></bml></act>')
    | 
    | function aFcnTruthTableAction_8()
    | 
    | % neutralHeadGaze
    | 
    | poseBML=encStr2Arr('<?xml version="1.0" ?><act><bml><gaze target="camera" sbm:time-hint="0.2"/></bml></act>')
  function gazeBML=boredGazeCompleteTable(bmlID):
    | function gazeBML=boredGazeCompleteTable(bmlID)
    | 
    | aVarTruthTableCondition_1 = false;
    | aVarTruthTableCondition_2 = false;
    | aVarTruthTableCondition_3 = false;
    | aVarTruthTableCondition_4 = false;
    | aVarTruthTableCondition_5 = false;
    | aVarTruthTableCondition_6 = false;
    | aVarTruthTableCondition_7 = false;
    | aVarTruthTableCondition_8 = false;
    | aVarTruthTableCondition_9 = false;
    | aVarTruthTableCondition_10 = false;
    | aVarTruthTableCondition_11 = false;
    | aVarTruthTableCondition_12 = false;
    | aVarTruthTableCondition_13 = false;
    | aVarTruthTableCondition_14 = false;
    | aVarTruthTableCondition_15 = false;
    | aVarTruthTableCondition_16 = false;
    | aVarTruthTableCondition_17 = false;
    | aVarTruthTableCondition_18 = false;
    | 
    | 
    | 
    | aVarTruthTableCondition_1 = logical(bmlID==1);
    | 
    | 
    | aVarTruthTableCondition_2 = logical(bmlID==2);
    | 
    | 
    | aVarTruthTableCondition_3 = logical(bmlID==3);
    | 
    | 
    | aVarTruthTableCondition_4 = logical(bmlID==4);
    | 
    | 
    | aVarTruthTableCondition_5 = logical(bmlID==5);
    | 
    | 
    | aVarTruthTableCondition_6 = logical(bmlID==6);
    | 
    | 
    | aVarTruthTableCondition_7 = logical(bmlID==7);
    | 
    | 
    | aVarTruthTableCondition_8 = logical(bmlID==8);
    | 
    | 
    | aVarTruthTableCondition_9 = logical(bmlID==9);
    | 
    | 
    | aVarTruthTableCondition_10 = logical(bmlID==10);
    | 
    | 
    | aVarTruthTableCondition_11 = logical(bmlID==11);
    | 
    | 
    | aVarTruthTableCondition_12 = logical(bmlID==12);
    | 
    | 
    | aVarTruthTableCondition_13 = logical(bmlID==13);
    | 
    | 
    | aVarTruthTableCondition_14 = logical(bmlID==14);
    | 
    | 
    | aVarTruthTableCondition_15 = logical(bmlID==15);
    | 
    | 
    | aVarTruthTableCondition_16 = logical(bmlID==16);
    | 
    | 
    | aVarTruthTableCondition_17 = logical(bmlID==17);
    | 
    | 
    | aVarTruthTableCondition_18 = logical(bmlID==18);
    | 
    | if (aVarTruthTableCondition_1)
    |     aFcnTruthTableAction_1();
    | elseif (aVarTruthTableCondition_2)
    |     aFcnTruthTableAction_2();
    | elseif (aVarTruthTableCondition_3)
    |     aFcnTruthTableAction_3();
    | elseif (aVarTruthTableCondition_4)
    |     aFcnTruthTableAction_4();
    | elseif (aVarTruthTableCondition_5)
    |     aFcnTruthTableAction_5();
    | elseif (aVarTruthTableCondition_6)
    |     aFcnTruthTableAction_6();
    | elseif (aVarTruthTableCondition_7)
    |     aFcnTruthTableAction_7();
    | elseif (aVarTruthTableCondition_8)
    |     aFcnTruthTableAction_8();
    | elseif (aVarTruthTableCondition_9)
    |     aFcnTruthTableAction_9();
    | elseif (aVarTruthTableCondition_10)
    |     aFcnTruthTableAction_10();
    | elseif (aVarTruthTableCondition_11)
    |     aFcnTruthTableAction_11();
    | elseif (aVarTruthTableCondition_12)
    |     aFcnTruthTableAction_12();
    | elseif (aVarTruthTableCondition_13)
    |     aFcnTruthTableAction_13();
    | elseif (aVarTruthTableCondition_14)
    |     aFcnTruthTableAction_14();
    | elseif (aVarTruthTableCondition_15)
    |     aFcnTruthTableAction_15();
    | elseif (aVarTruthTableCondition_16)
    |     aFcnTruthTableAction_16();
    | elseif (aVarTruthTableCondition_17)
    |     aFcnTruthTableAction_25();
    | elseif (aVarTruthTableCondition_18)
    |     aFcnTruthTableAction_26();
    | else % Default
    |     aFcnTruthTableAction_1();
    | end
    | 
    | function aFcnTruthTableAction_1()
    | 
    | % LeftS
    | 
    | gazeBML=encStr2Arr('<?xml version="1.0" ?><act><bml><gaze angle="12" direction="LEFT" sbm:joint-range="EYES" target="camera"/></bml></act>')
    | 
    | function aFcnTruthTableAction_2()
    | 
    | % RightS
    | 
    | gazeBML=encStr2Arr('<?xml version="1.0" ?><act><bml><gaze angle="12" direction="RIGHT" sbm:joint-range="EYES" target="camera"/></bml></act>')
    | 
    | function aFcnTruthTableAction_3()
    | 
    | % UpS
    | 
    | gazeBML=encStr2Arr('<?xml version="1.0" ?><act><bml><gaze angle="12" direction="UP" sbm:joint-range="EYES" target="camera"/></bml></act>')
    | 
    | function aFcnTruthTableAction_4()
    | 
    | % DownS
    | 
    | gazeBML=encStr2Arr('<?xml version="1.0" ?><act><bml><gaze angle="12" direction="DOWN" sbm:joint-range="EYES" target="camera"/></bml></act>')
    | 
    | function aFcnTruthTableAction_5()
    | 
    | % UpLeftS
    | 
    | gazeBML=encStr2Arr('<?xml version="1.0" ?><act><bml><gaze angle="12" direction="UPLEFT" sbm:joint-range="EYES" target="camera"/></bml></act>')
    | 
    | function aFcnTruthTableAction_6()
    | 
    | % UpRightS
    | 
    | gazeBML=encStr2Arr('<?xml version="1.0" ?><act><bml><gaze angle="12" direction="UPRIGHT" sbm:joint-range="EYES" target="camera"/></bml></act>')
    | 
    | function aFcnTruthTableAction_7()
    | 
    | % DownLeftS
    | 
    | gazeBML=encStr2Arr('<?xml version="1.0" ?><act><bml><gaze angle="12" direction="DOWNLEFT" sbm:joint-range="EYES" target="camera"/></bml></act>')
    | 
    | function aFcnTruthTableAction_8()
    | 
    | % DownRightS
    | 
    | gazeBML=encStr2Arr('<?xml version="1.0" ?><act><bml><gaze angle="12" direction="DOWNRIGHT" sbm:joint-range="EYES" target="camera"/></bml></act>')
    | 
    | function aFcnTruthTableAction_9()
    | 
    | % Down
    | 
    | gazeBML=encStr2Arr('<?xml version="1.0" ?><act><bml><gaze direction="DOWN" sbm:joint-range="EYES NECK" sbm:time-hint="0.15" target="camera"/></bml></act>')
    | 
    | function aFcnTruthTableAction_10()
    | 
    | % Downleft
    | 
    | gazeBML=encStr2Arr('<?xml version="1.0" ?><act><bml><gaze direction="DOWNLEFT" sbm:joint-range="EYES NECK" sbm:time-hint="0.15" target="camera"/></bml></act>')
    | 
    | function aFcnTruthTableAction_11()
    | 
    | % Downright
    | 
    | gazeBML=encStr2Arr('<?xml version="1.0" ?><act><bml><gaze direction="DOWNRIGHT" sbm:joint-range="EYES NECK" sbm:time-hint="0.15" target="camera"/></bml></act>')
    | 
    | function aFcnTruthTableAction_12()
    | 
    | % Upright
    | 
    | gazeBML=encStr2Arr('<?xml version="1.0" ?><act><bml><gaze direction="UPRIGHT" sbm:joint-range="EYES NECK" sbm:time-hint="0.15" target="camera"/></bml></act>')
    | 
    | function aFcnTruthTableAction_13()
    | 
    | % Upleft
    | 
    | gazeBML=encStr2Arr('<?xml version="1.0" ?><act><bml><gaze direction="UPLEFT" sbm:joint-range="EYES NECK" sbm:time-hint="0.15" target="camera"/></bml></act>')
    | 
    | function aFcnTruthTableAction_14()
    | 
    | % Up
    | 
    | gazeBML=encStr2Arr('<?xml version="1.0" ?><act><bml><gaze direction="UP" sbm:joint-range="EYES NECK" sbm:time-hint="0.15" target="camera"/></bml></act>')
    | 
    | function aFcnTruthTableAction_15()
    | 
    | % Right
    | 
    | gazeBML=encStr2Arr('<?xml version="1.0" ?><act><bml><gaze direction="RIGHT" sbm:joint-range="EYES NECK" sbm:time-hint="0.15" target="camera"/></bml></act>')
    | 
    | function aFcnTruthTableAction_16()
    | 
    | % LEFT
    | 
    | gazeBML=encStr2Arr('<?xml version="1.0" ?><act><bml><gaze direction="LEFT" sbm:joint-range="EYES NECK" sbm:time-hint="0.15" target="camera"/></bml></act>')
    | 
    | function aFcnTruthTableAction_17()
    | 
    | % DownLeftSN
    | 
    | gazeBML=encStr2Arr('<?xml version="1.0" ?><act><bml><gaze angle="12" direction="LEFT" sbm:joint-range="NECK" sbm:time-hint="0.15" target="camera"/></bml></act>')
    | 
    | function aFcnTruthTableAction_18()
    | 
    | % DownRightSN
    | 
    | gazeBML=encStr2Arr('<?xml version="1.0" ?><act><bml><gaze angle="12" direction="RIGHT" sbm:joint-range="NECK" sbm:time-hint="0.15" target="camera"/></bml></act>')
    | 
    | function aFcnTruthTableAction_19()
    | 
    | % DownUpSN
    | 
    | gazeBML=encStr2Arr('<?xml version="1.0" ?><act><bml><gaze angle="12" direction="UP" sbm:joint-range="HEAD CHEST" sbm:time-hint="0.3" target="camera"/></bml></act>')
    | 
    | function aFcnTruthTableAction_20()
    | 
    | % DownDownSN
    | 
    | gazeBML=encStr2Arr('<?xml version="1.0" ?><act><bml><gaze angle="12" direction="DOWN" sbm:joint-range="NECK" sbm:time-hint="0.15" target="camera"/></bml></act>')
    | 
    | function aFcnTruthTableAction_21()
    | 
    | % DownUPLEFTSN
    | 
    | gazeBML=encStr2Arr('<?xml version="1.0" ?><act><bml><gaze angle="12" direction="UPLEFT" sbm:joint-range="NECK" sbm:time-hint="0.15" target="camera"/></bml></act>')
    | 
    | function aFcnTruthTableAction_22()
    | 
    | % DownUPRIGHTSN
    | 
    | gazeBML=encStr2Arr('<?xml version="1.0" ?><act><bml><gaze angle="12" direction="UPRIGHT" sbm:joint-range="NECK" sbm:time-hint="0.15" target="camera"/></bml></act>')
    | 
    | function aFcnTruthTableAction_23()
    | 
    | % DownDOWNLEFTSN
    | 
    | gazeBML=encStr2Arr('<?xml version="1.0" ?><act><bml><gaze angle="12" direction="DOWNLEFT" sbm:joint-range="NECK" sbm:time-hint="0.15" target="camera"/></bml></act>')
    | 
    | function aFcnTruthTableAction_24()
    | 
    | % DownDOWNRightSN
    | 
    | gazeBML=encStr2Arr('<?xml version="1.0" ?><act><bml><gaze angle="12" direction="DOWNRIGHT" sbm:joint-range="NECK" sbm:time-hint="0.15" target="camera"/></bml></act>')
    | 
    | function aFcnTruthTableAction_25()
    | 
    | % blink
    | 
    | gazeBML=encStr2Arr('<?xml version="1.0" ?><act><bml><face type="FACS" side="BOTH" au="45" amount="0.5" /></bml></act>')
    | 
    | function aFcnTruthTableAction_26()
    | 
    | % eyebrowUp
    | 
    | gazeBML=encStr2Arr('<?xml version="1.0" ?><act><bml><face amount="0.3" au="1" stroke="3" relax="4" end="6" side="BOTH" start="0" type="facs"/><face amount="0.8"  stroke="3" relax="4" au="2" end="6" side="BOTH" start="0" type="facs"/></bml></act>')
